simulink model "untitled1"  (R2022b)
settings: Solver=VariableStepAuto  StartTime=0.0  StopTime=10.0  RelTol=1e-3
settings Model: DataDictionary=BusSystem.sldd  Creator=Robert  LastModifiedBy=Robert

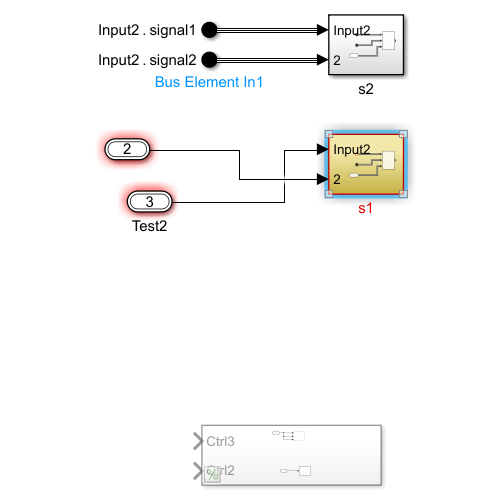
[thumbnail: Simulink's stored preview of the top-level diagram]
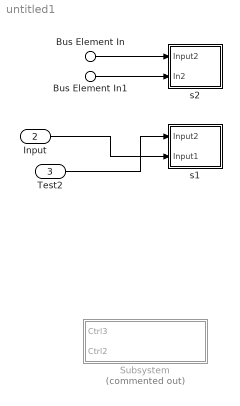
== system untitled1 ==
  Bus Element In : Inport  PortName=Input2  Element=signal1
  Bus Element In1 : Inport  PortName=Input2  Element=signal2
  Input : Inport  Port=2  OutDataTypeStr=Bus: bus8
  Test2 : Inport  Port=3  OutDataTypeStr=Bus: bus10
  Subsystem : Subsystem  Commented=on
  s1 : Subsystem
  s2 : Subsystem
  wires:
  Bus Element In/1 -> s2/1(Input2)
  Bus Element In1/1 -> s2/2(In2)
  Input/1 -> s1/2(Input1)
  Test2/1 -> s1/1(Input2)

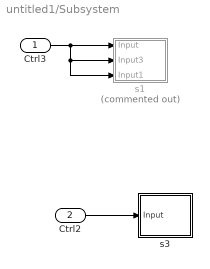
== system untitled1/Subsystem ==
  Ctrl3 : Inport
  Ctrl2 : Inport  Port=2
  s1 : Subsystem  Commented=on
  s3 : Subsystem
  wires:
  Ctrl3/1 -> s1/3(Input1), s1/2(Input3), s1/1(Input)
  Ctrl2/1 -> s3/1(Input)

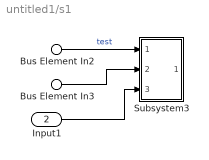
== system untitled1/s1 ==
  Bus Element In3 : Inport  PortName=Input2  Element=mul1
  Bus Element In2 : Inport  PortName=Input2  Element=mult2
  Input1 : Inport  Port=2
  Subsystem3 : Subsystem
  wires:
  Input1/1 -> Subsystem3/3(Input2)
  Bus Element In3/1 -> Subsystem3/2(In2)
  Bus Element In2/1 -> Subsystem3/1(In1)  "test"

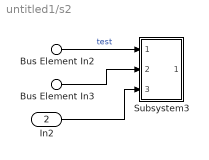
== system untitled1/s2 ==
  Bus Element In3 : Inport  PortName=Input2  Element=mul1
  Bus Element In2 : Inport  PortName=Input2  Element=mult2
  In2 : Inport  Port=2
  Subsystem3 : Subsystem
  wires:
  Bus Element In2/1 -> Subsystem3/1(In1)  "test"
  Bus Element In3/1 -> Subsystem3/2(In2)
  In2/1 -> Subsystem3/3(Input2)

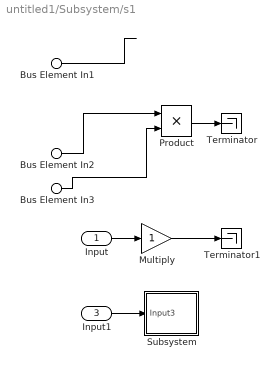
== system untitled1/Subsystem/s1 ==
  Input : Inport
  Bus Element In1 : Inport  Port=2  PortName=Input3  Element=mul4
  Bus Element In2 : Inport  Port=2  PortName=Input3  Element=mul1
  Bus Element In3 : Inport  Port=2  PortName=Input3  Element=mul1
  Input1 : Inport  Port=3
  Multiply : Gain
  Product : Product
  Subsystem : Subsystem
  Terminator : Terminator
  Terminator1 : Terminator
  wires:
  Input/1 -> Multiply/1
  Bus Element In1/1 -> ?
  Bus Element In2/1 -> Product/1
  Bus Element In3/1 -> Product/2
  Product/1 -> Terminator/1
  Multiply/1 -> Terminator1/1
  Input1/1 -> Subsystem/1(Input3)

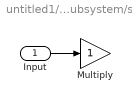
== system untitled1/Subsystem/s3 ==
  Input : Inport
  Multiply : Gain
  wires:
  Input/1 -> Multiply/1

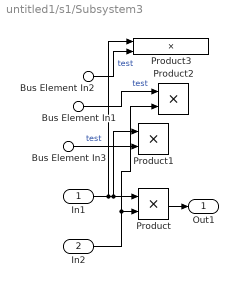
== system untitled1/s1/Subsystem3 ==
  In1 : Inport
  In2 : Inport  Port=2
  Bus Element In2 : Inport  Port=3  PortName=Input2  Element=mult2
  Bus Element In1 : Inport  Port=3  PortName=Input2  Element=mult1
  Bus Element In3 : Inport  Port=3  PortName=Input2  Element=mult3
  Product{,1..3} (4 alike) : Product
  Out1 : Outport
  wires:
  Bus Element In3/1 -> Product1/2  "test"
  Bus Element In1/1 -> Product2/1  "test"
  Bus Element In2/1 -> Product3/2  "test"
  In2/1 -> Product/2, Product2/2
  In1/1 -> Product/1, Product1/1, Product3/1
  Product/1 -> Out1/1

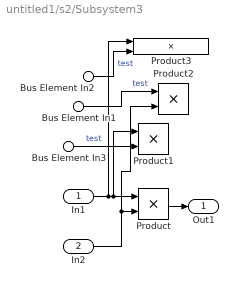
== system untitled1/s2/Subsystem3 ==
  In1 : Inport
  In2 : Inport  Port=2
  Bus Element In2 : Inport  Port=3  PortName=Input2  Element=mult2
  Bus Element In1 : Inport  Port=3  PortName=Input2  Element=mult1
  Bus Element In3 : Inport  Port=3  PortName=Input2  Element=mult3
  Product{,1..3} (4 alike) : Product
  Out1 : Outport
  wires:
  Product/1 -> Out1/1
  In1/1 -> Product3/1, Product1/1, Product/1
  In2/1 -> Product2/2, Product/2
  Bus Element In2/1 -> Product3/2  "test"
  Bus Element In1/1 -> Product2/1  "test"
  Bus Element In3/1 -> Product1/2  "test"

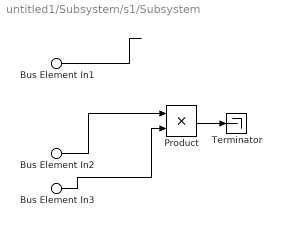
== system untitled1/Subsystem/s1/Subsystem ==
  Bus Element In1 : Inport  PortName=Input3  Element=mul4
  Bus Element In2 : Inport  PortName=Input3  Element=mul1
  Bus Element In3 : Inport  PortName=Input3  Element=mul1
  Product : Product
  Terminator : Terminator
  wires:
  Bus Element In3/1 -> Product/2
  Bus Element In2/1 -> Product/1
  Bus Element In1/1 -> ?
  Product/1 -> Terminator/1
